simulink model "MLP_networks"  (Simulink 7.7)
settings: Solver=ode45  StartTime=0.0  StopTime=10.0  RelTol=1e-3
libraries: neural x1629
(part 13 of 39)

== system MLP_networks/net_col_c_d_2_4/Layer 2/LW{2,1} ==
  "ad{2,1}" : Inport  PortDimensions=30
      mask Display: e = 0.06;c1 = [120 230 180]/255;c2 = ([120 230 180]+0)/(256+128);c3 = ([120 230 180]+128)/(256+128);patch([0 1 1 0],[0 0 1 1],c1);patch([0 1 1 1-e 1-e 0+e],[0 0 1 1-e 0+e 0+e],c2);patch([0 0 1 1-e 0+e 0+e],[0 1 1 1-e 1-e 0+e],c3);plot([0 1 1 0 0],[0 0 1 1 0]);
  "IW{2,1}(1,:)'" : Constant  Value=[-0.086739905279401591;-0.34352499863211877;0.41397198976248467;0.43609623522289326;0.083435443764242001;0.19327035793616087;-0.27874403632422867;-0.11777803771657309;-0.023646706701705794;0.32594090440830897;-0.12873398528261154;0.33611135005815379;0.40852985787112106;-0.33466057721896658;-0.052474886443023012;0.43264924815576428;0.12741649927597465;0.03311259969224789;-0.19344074611037179;0.24350359634959076;-0.45438070656869112;0.40836563164644157;0.4762716734952942;-0.27838513598564113;-0.065634489210694244;-0.29128069108023635;0.25511712952102317;-0.46499974373678382;-0.0088992625430886971;0.13908009278308667]
      mask Display: e = 0.06;c1 = [120 150 230]/255;c2 = ([120 150 230]+0)/383;c3 = ([120 150 230]+128)/383;patch([0 1 1 0],[0 0 1 1],c1);patch([0 1 1 1-e 1-e 0+e],[0 0 1 1-e 0+e 0+e],c2);patch([0 0 1 1-e 0+e 0+e],[0 1 1 1-e 1-e 0+e],c3);plot([0 1 1 0 0],[0 0 1 1 0]);disp('weights');
  "IW{2,1}(10,:)'" : Constant  Value=[-0.36729620765024679;0.0050898962860818709;-0.0468691936394676;0.1253497976658039;0.47105014411088103;0.0033716376305642725;-0.41138077394803518;-0.32349762312197461;0.39546656477867215;-0.22070804075098249;0.042861658999594557;-0.12681144224424798;-0.25039111248890011;-0.3712654210908593;0.56958995394778955;-0.044483129058483888;-0.34197575262972091;0.17028025717551185;0.1085468634386007;0.14691948303331084;-0.19893228667253338;0.43968182733407096;-0.53408102802366886;0.17496913310039999;0.097757521509979323;0.33217818846497571;-0.045631385768622072;-0.37542745057039434;0.33335878174126277;-0.068873205774028126]
      mask Display: e = 0.06;c1 = [120 150 230]/255;c2 = ([120 150 230]+0)/383;c3 = ([120 150 230]+128)/383;patch([0 1 1 0],[0 0 1 1],c1);patch([0 1 1 1-e 1-e 0+e],[0 0 1 1-e 0+e 0+e],c2);patch([0 0 1 1-e 0+e 0+e],[0 1 1 1-e 1-e 0+e],c3);plot([0 1 1 0 0],[0 0 1 1 0]);disp('weights');
  "IW{2,1}(11,:)'" : Constant  Value=[-0.21023796895427466;0.21178254562760829;-0.1516673968740547;0.2773361318766529;0.012215682673962412;-0.48546667397653748;-0.18369601082146786;-0.26072759710949656;-0.053448210306775074;0.20320759307683936;0.15049891040467875;0.10455567206696842;0.4429239128696621;-0.20191752051219272;0.29857936146071512;0.48716984305870775;-0.21868844150185676;0.39089943245601361;-0.38722549529227124;0.20420721060355676;-0.58146629375206382;-0.14308677037043016;0.092893812514471041;-0.30523259519614931;-0.29641244502780845;0.055601417546032407;-0.14166216047879499;0.39149809987544448;0.3731245822311216;-0.083752309554754018]
      mask Display: e = 0.06;c1 = [120 150 230]/255;c2 = ([120 150 230]+0)/383;c3 = ([120 150 230]+128)/383;patch([0 1 1 0],[0 0 1 1],c1);patch([0 1 1 1-e 1-e 0+e],[0 0 1 1-e 0+e 0+e],c2);patch([0 0 1 1-e 0+e 0+e],[0 1 1 1-e 1-e 0+e],c3);plot([0 1 1 0 0],[0 0 1 1 0]);disp('weights');
  "IW{2,1}(12,:)'" : Constant  Value=[-0.22221752783866594;-0.463286764183786;0.32012275560695169;0.25096255632346381;0.0050231260198129787;-0.41543038790111159;-0.042578931985107822;-0.229325715588483;-0.094594039183964918;0.12192301882377349;-0.2291642495939753;0.34948087306916753;-0.22411941369390356;-0.25980901333444251;0.0099306671826360823;-0.21571241200028116;-0.3003090801392887;0.36235995289088319;0.41424763108456042;0.4549194867057913;-0.38526533593013734;-0.027743054382739805;-0.20900585233406158;-0.35337276927947708;0.11255897424267725;-0.039132173089780509;-0.42824103440953348;0.44315723034418508;0.084105476144599511;0.37576155528745614]
      mask Display: e = 0.06;c1 = [120 150 230]/255;c2 = ([120 150 230]+0)/383;c3 = ([120 150 230]+128)/383;patch([0 1 1 0],[0 0 1 1],c1);patch([0 1 1 1-e 1-e 0+e],[0 0 1 1-e 0+e 0+e],c2);patch([0 0 1 1-e 0+e 0+e],[0 1 1 1-e 1-e 0+e],c3);plot([0 1 1 0 0],[0 0 1 1 0]);disp('weights');
  "IW{2,1}(13,:)'" : Constant  Value=[0.26664690956162634;0.18588211338743232;-0.51074478099671949;-0.23272464385698416;-0.11789865989217188;0.33770596273549025;-0.41543902149946016;-0.20325083039795819;0.21359489198140075;0.23771981850878229;-0.10782260011209335;-0.4560526783866341;-0.49243186311351428;0.35164195674675991;0.091680564545084595;-0.1416316671420981;0.090346906082689124;-0.26101314139369514;-0.070749610911415614;-0.40337304681422642;0.11262128161825263;-0.27525094149576945;-0.12145424331596209;-0.3151042810855188;-0.12176588049624475;-0.40594084401160607;0.40726344059532144;-0.13387975813296663;0.48118452093616576;0.27020875321167304]
      mask Display: e = 0.06;c1 = [120 150 230]/255;c2 = ([120 150 230]+0)/383;c3 = ([120 150 230]+128)/383;patch([0 1 1 0],[0 0 1 1],c1);patch([0 1 1 1-e 1-e 0+e],[0 0 1 1-e 0+e 0+e],c2);patch([0 0 1 1-e 0+e 0+e],[0 1 1 1-e 1-e 0+e],c3);plot([0 1 1 0 0],[0 0 1 1 0]);disp('weights');
  "IW{2,1}(14,:)'" : Constant  Value=[0.34980934949483533;0.1234860655908767;0.41357778903144787;0.052540691627614988;0.25997646810356406;0.019550504650392903;-0.41112577725337546;-0.004004284700734397;0.20936217792212469;0.33508267363697175;-0.20605229449470713;0.30248198819108618;0.15830807524143486;-0.25625975309585886;-0.28171785254204545;0.39217753159778523;-0.39365391187201221;0.34365095949680785;0.179703187893896;0.39471168575822613;0.0051157792018336453;-0.09392142748098764;0.24890008564234903;0.27724910625266452;0.3897128187753453;0.43225990952346627;-0.4134253832902795;0.34873671936583894;-0.16432440790350927;-0.26930883733609756]
      mask Display: e = 0.06;c1 = [120 150 230]/255;c2 = ([120 150 230]+0)/383;c3 = ([120 150 230]+128)/383;patch([0 1 1 0],[0 0 1 1],c1);patch([0 1 1 1-e 1-e 0+e],[0 0 1 1-e 0+e 0+e],c2);patch([0 0 1 1-e 0+e 0+e],[0 1 1 1-e 1-e 0+e],c3);plot([0 1 1 0 0],[0 0 1 1 0]);disp('weights');
  "IW{2,1}(15,:)'" : Constant  Value=[0.10756034167331048;0.027268277800464581;0.23872494323237675;-0.26516481299813138;0.26000758623086434;-0.39846704436064129;-0.27015200960985691;-0.44604290248752793;0.42864135743800169;-0.4469329110749522;0.16848395781183378;-0.051220464237963677;0.086400763208768563;-0.10129868161474533;-0.026199243651805027;0.30436336508280776;-0.25002859827495977;-0.0072896443892497232;0.35355014668734541;0.37370190785436924;0.26582471435491495;-0.043249001392198672;0.44844689361690387;0.35439045498470667;0.21055831758031823;-0.27598099185526553;-0.35847563137517258;0.33563489845674022;0.3657385019059855;0.33310742263125259]
      mask Display: e = 0.06;c1 = [120 150 230]/255;c2 = ([120 150 230]+0)/383;c3 = ([120 150 230]+128)/383;patch([0 1 1 0],[0 0 1 1],c1);patch([0 1 1 1-e 1-e 0+e],[0 0 1 1-e 0+e 0+e],c2);patch([0 0 1 1-e 0+e 0+e],[0 1 1 1-e 1-e 0+e],c3);plot([0 1 1 0 0],[0 0 1 1 0]);disp('weights');
  "IW{2,1}(16,:)'" : Constant  Value=[-0.22297684824986103;-0.35714462966301846;0.48875156904773898;-0.04051019970576434;0.41685592475144728;-0.12244765379847856;-0.40779118540112924;0.023197515559235875;-0.045272172969816532;-0.023956146090705222;-0.44229605346214801;-0.10538638233096333;-0.30887898599700275;-0.40889553293161374;0.071952147052590343;-0.48675313221945821;-0.35492176719265267;-0.13320271136704864;0.25380506446655143;0.19576911876540612;0.15700698328941776;0.48317096404336252;0.31386156255509157;-0.29817432668524568;-0.23166046191463932;0.2076614117377503;-0.065995897941546824;-0.4446390086503117;0.10384621552539763;-0.10499763342719416]
      mask Display: e = 0.06;c1 = [120 150 230]/255;c2 = ([120 150 230]+0)/383;c3 = ([120 150 230]+128)/383;patch([0 1 1 0],[0 0 1 1],c1);patch([0 1 1 1-e 1-e 0+e],[0 0 1 1-e 0+e 0+e],c2);patch([0 0 1 1-e 0+e 0+e],[0 1 1 1-e 1-e 0+e],c3);plot([0 1 1 0 0],[0 0 1 1 0]);disp('weights');
  "IW{2,1}(17,:)'" : Constant  Value=[-0.20818659317735247;0.37291404688386326;-0.066412472318293309;0.23880592375907964;-0.17470240698411357;0.36274967181515411;-0.29500641736352323;0.3612460607052741;0.35349882887855227;0.50867004947603289;-0.24957816422824536;-0.37050881703534111;-0.17894190937801782;-0.4020952164867897;0.16763586618568879;-0.34269716360850005;0.31470217864282929;0.16211539237220335;0.35180618314252515;-0.052516647446877403;0.050581096159848335;0.039637997646489689;-0.2790044063742475;0.21372505912316375;0.087182966437931317;0.24205750316420507;-0.49727888668810799;-0.0062618082043166736;-0.66180921273073823;-0.15908637712630638]
      mask Display: e = 0.06;c1 = [120 150 230]/255;c2 = ([120 150 230]+0)/383;c3 = ([120 150 230]+128)/383;patch([0 1 1 0],[0 0 1 1],c1);patch([0 1 1 1-e 1-e 0+e],[0 0 1 1-e 0+e 0+e],c2);patch([0 0 1 1-e 0+e 0+e],[0 1 1 1-e 1-e 0+e],c3);plot([0 1 1 0 0],[0 0 1 1 0]);disp('weights');
  "IW{2,1}(18,:)'" : Constant  Value=[-0.063784427387764658;-0.32883070779687101;-0.48245120779581252;0.39650567321388691;-0.44937991772281205;0.01898057625759408;-0.12935469257041271;0.39546243145334697;-0.22112563100831639;0.38159471583348348;0.47658380504876108;0.29114272831383531;0.081150065748367251;-0.35952532056727365;0.43105590479120115;0.36632351247334227;0.088108073808608592;-0.37722671859528067;0.12912619522745261;0.23488410715253483;0.10081022555742715;0.11318476809914328;0.37249559297773699;0.22920497316165944;-0.089689746006884327;-0.053868567690606883;-0.37766729562412882;-0.35274036741954445;0.073527138309710388;-0.10041159535850687]
      mask Display: e = 0.06;c1 = [120 150 230]/255;c2 = ([120 150 230]+0)/383;c3 = ([120 150 230]+128)/383;patch([0 1 1 0],[0 0 1 1],c1);patch([0 1 1 1-e 1-e 0+e],[0 0 1 1-e 0+e 0+e],c2);patch([0 0 1 1-e 0+e 0+e],[0 1 1 1-e 1-e 0+e],c3);plot([0 1 1 0 0],[0 0 1 1 0]);disp('weights');
  "IW{2,1}(19,:)'" : Constant  Value=[0.19336196700834571;0.26744725560522559;-0.12860710197058553;0.31928174667930265;-0.070050044733280872;0.23283023634842093;0.30818323009661364;0.22289340702256244;-0.040112984385321182;0.46550220777364704;-0.35005738655757873;0.47597538337899226;-0.44170921923744139;-0.26572842897223375;-0.34489183248480759;0.18140277900820642;0.28607657081867038;0.086576963143464039;-0.3072812531424518;-0.034491965720857221;-0.39374044579926959;-0.18234841076921057;-0.35726304605837306;0.52328133768006635;0.21393030940681942;-0.11424070367808993;0.023196839579096535;0.15293831083094575;-0.30406146637276343;0.42953594576905829]
      mask Display: e = 0.06;c1 = [120 150 230]/255;c2 = ([120 150 230]+0)/383;c3 = ([120 150 230]+128)/383;patch([0 1 1 0],[0 0 1 1],c1);patch([0 1 1 1-e 1-e 0+e],[0 0 1 1-e 0+e 0+e],c2);patch([0 0 1 1-e 0+e 0+e],[0 1 1 1-e 1-e 0+e],c3);plot([0 1 1 0 0],[0 0 1 1 0]);disp('weights');
  "IW{2,1}(2,:)'" : Constant  Value=[-0.31476253520435571;-0.1138264490805047;-0.45036209335075572;0.2714809849441942;-0.18735671368056603;0.43408018666630871;-0.071620807727931404;0.048980335818204206;0.43751144967020755;0.020604521452307876;-0.10660971195039906;-0.3560330087569426;0.020071737319517006;-0.18091744791693601;0.40865545415885268;0.44681513013327728;0.38130042131451752;-0.23103110817028119;-0.42668382247905429;-0.39432400289217451;-0.22914394412555436;0.34667621785082403;-0.20755805619700282;0.057989851918950258;0.36069318624763025;0.34715274095295884;0.24150077728754232;0.2229140129936108;0.1240409175129034;-0.16506729455336752]
      mask Display: e = 0.06;c1 = [120 150 230]/255;c2 = ([120 150 230]+0)/383;c3 = ([120 150 230]+128)/383;patch([0 1 1 0],[0 0 1 1],c1);patch([0 1 1 1-e 1-e 0+e],[0 0 1 1-e 0+e 0+e],c2);patch([0 0 1 1-e 0+e 0+e],[0 1 1 1-e 1-e 0+e],c3);plot([0 1 1 0 0],[0 0 1 1 0]);disp('weights');
  "IW{2,1}(20,:)'" : Constant  Value=[0.33658701609073133;-0.17880093932274299;0.28437477283972262;0.39176322624983256;0.34816982312398603;-0.27806344079324408;-0.13224436335612005;0.23658674697646723;0.31463988161876533;0.23333367558291757;-0.20140728285472401;0.38983013905004149;-0.30351607692150379;-0.28449349935494206;-0.20626698506988783;-0.35004568799273844;-0.12100694505081969;0.21073444675825728;0.4293641950214887;-0.079932739921778573;-0.16946655759443563;-0.41523238613031477;-0.22719246897086262;0.11304598071208617;-0.1468262990874139;-0.50528490331397169;-0.43436092951156996;-0.40874554765229931;-0.15439640651095748;-0.10139444109459227]
      mask Display: e = 0.06;c1 = [120 150 230]/255;c2 = ([120 150 230]+0)/383;c3 = ([120 150 230]+128)/383;patch([0 1 1 0],[0 0 1 1],c1);patch([0 1 1 1-e 1-e 0+e],[0 0 1 1-e 0+e 0+e],c2);patch([0 0 1 1-e 0+e 0+e],[0 1 1 1-e 1-e 0+e],c3);plot([0 1 1 0 0],[0 0 1 1 0]);disp('weights');
  "IW{2,1}(21,:)'" : Constant  Value=[0.18698793822477749;0.44710802080556572;0.055362238215656438;-0.10315370156659233;-0.093547650109901181;0.48144329663092722;-0.3487454699215734;-0.3357544725505629;-0.52892778597397039;-0.15570016555093408;0.019344232566923886;-0.057459364801196039;-0.10882588337634393;-0.13026152839250427;0.31546914479780114;-0.54184132761413528;-0.20814735027442335;-0.50581397740701151;0.066142940955517926;-0.073780813119728506;-0.019554590542029657;0.3076647815515357;-0.51496038974850633;-0.20453340312828328;0.46321035495375734;0.12406975452781493;-0.025668149130415988;-0.16131670207754562;0.40620666634841929;-0.27237136393892403]
      mask Display: e = 0.06;c1 = [120 150 230]/255;c2 = ([120 150 230]+0)/383;c3 = ([120 150 230]+128)/383;patch([0 1 1 0],[0 0 1 1],c1);patch([0 1 1 1-e 1-e 0+e],[0 0 1 1-e 0+e 0+e],c2);patch([0 0 1 1-e 0+e 0+e],[0 1 1 1-e 1-e 0+e],c3);plot([0 1 1 0 0],[0 0 1 1 0]);disp('weights');
  "IW{2,1}(22,:)'" : Constant  Value=[-0.30183550782893204;0.18593285110881588;0.051690249772538249;0.42467534385490119;0.12917866311309761;-0.46077057472685201;0.023141069862614577;0.14345569870191224;-0.063414483521242584;0.48237058045684522;-0.055378234308140824;0.29182892206326488;0.42334775055828106;0.33457671039397663;0.43955355934047158;-0.0030498102862665721;0.34715523973677864;-0.37986667441238248;0.29783656860234109;0.12222242933619888;-0.044754535324555048;0.42544662656884691;-0.16407975067525937;-0.15912099798763263;-0.45811143300484625;-0.39655212784155747;0.31857894815139959;-0.23994535950314261;0.23029394329595129;0.10679840935171044]
      mask Display: e = 0.06;c1 = [120 150 230]/255;c2 = ([120 150 230]+0)/383;c3 = ([120 150 230]+128)/383;patch([0 1 1 0],[0 0 1 1],c1);patch([0 1 1 1-e 1-e 0+e],[0 0 1 1-e 0+e 0+e],c2);patch([0 0 1 1-e 0+e 0+e],[0 1 1 1-e 1-e 0+e],c3);plot([0 1 1 0 0],[0 0 1 1 0]);disp('weights');
  "IW{2,1}(23,:)'" : Constant  Value=[0.053371052201615247;-0.49742073003002413;-0.3599435655909598;0.16330570695765617;-0.41532433512319111;0.09863006949822134;-0.29326825977264376;0.30729900401793153;-0.065949061443200174;0.11198886134314458;0.36820832074642851;-0.24578993140959082;-0.15348153563585035;0.48631579535407221;0.13138601761928562;0.1266852664445573;0.14448148795735102;0.51816404532104388;0.21273550099709346;0.40532426732531829;0.14530829635166378;-0.37547464479146891;-0.39977913170225465;-0.17169438892309066;0.053399449589075901;0.36049043906111888;-0.18142893811318006;0.42052136186239569;0.18973264143336227;0.0041478850787327456]
      mask Display: e = 0.06;c1 = [120 150 230]/255;c2 = ([120 150 230]+0)/383;c3 = ([120 150 230]+128)/383;patch([0 1 1 0],[0 0 1 1],c1);patch([0 1 1 1-e 1-e 0+e],[0 0 1 1-e 0+e 0+e],c2);patch([0 0 1 1-e 0+e 0+e],[0 1 1 1-e 1-e 0+e],c3);plot([0 1 1 0 0],[0 0 1 1 0]);disp('weights');
  "IW{2,1}(24,:)'" : Constant  Value=[0.20516641930919408;-0.13518158187186338;0.0031559816953125831;0.18139980194621383;-0.54341365942738007;0.33949462411693088;0.10313907071790988;0.31393660081584912;0.11321227617715977;0.045980862742651681;0.27200974181943832;0.67565470147675843;-0.14522217595114961;0.51602354093719782;-0.14943402842186573;0.58352681264601935;-0.10609970694290385;-0.0058408385127818952;-0.27600492769484047;-0.068484010904123274;0.098456691211598016;-0.17902535749425891;-0.00037140347666213828;-0.23887433643879744;-0.057275554320067604;-0.50549685308164283;0.46414337205761558;0.10624528725808427;0.10579439676794743;0.15549185179355696]
      mask Display: e = 0.06;c1 = [120 150 230]/255;c2 = ([120 150 230]+0)/383;c3 = ([120 150 230]+128)/383;patch([0 1 1 0],[0 0 1 1],c1);patch([0 1 1 1-e 1-e 0+e],[0 0 1 1-e 0+e 0+e],c2);patch([0 0 1 1-e 0+e 0+e],[0 1 1 1-e 1-e 0+e],c3);plot([0 1 1 0 0],[0 0 1 1 0]);disp('weights');
  "IW{2,1}(25,:)'" : Constant  Value=[0.34729406478959007;0.24899528893076581;0.38975618702404735;-0.43370060705451807;0.43967599939440211;0.24714052363443123;-0.23516138628203193;0.27112310701103942;0.30747614819565189;-0.25901471912936047;0.066960381916171249;0.021109088740329799;0.36800329396956483;-0.33773092533269283;0.16585516170887771;-0.39913557490327317;0.422381088012171;0.38751406788119919;-0.28623287820901655;-0.18588164855613096;0.16437778958045182;0.33801033214529363;-0.14353924983108626;-0.27136982002342719;-0.18588379207432654;-0.19026604050441728;0.43711302651380946;0.082818735914955685;0.10823163927324558;0.17381563706576]
      mask Display: e = 0.06;c1 = [120 150 230]/255;c2 = ([120 150 230]+0)/383;c3 = ([120 150 230]+128)/383;patch([0 1 1 0],[0 0 1 1],c1);patch([0 1 1 1-e 1-e 0+e],[0 0 1 1-e 0+e 0+e],c2);patch([0 0 1 1-e 0+e 0+e],[0 1 1 1-e 1-e 0+e],c3);plot([0 1 1 0 0],[0 0 1 1 0]);disp('weights');
  "IW{2,1}(26,:)'" : Constant  Value=[0.39572013934362721;0.21877832829196214;-0.15198346332651508;0.42066807388437649;0.31599505644468512;0.15381761781263398;0.14191037298792222;-0.025831073713321617;-0.15017548056642216;0.094845571844094187;-0.46918736211706985;-0.24436647216383825;0.14124572797964732;-0.27098572544577526;-0.48977172048525852;-0.17053071487204099;-0.21764468329733291;0.55221642220574907;-0.48813591066651452;-0.14388962884454987;0.21413565468843948;0.01795983414699797;0.3500296082403242;-0.046075493068468559;0.023259972562694051;-0.16960957564902857;0.34946590680847733;-0.32493567344175694;-0.79675058574351276;-0.040157404112677854]
      mask Display: e = 0.06;c1 = [120 150 230]/255;c2 = ([120 150 230]+0)/383;c3 = ([120 150 230]+128)/383;patch([0 1 1 0],[0 0 1 1],c1);patch([0 1 1 1-e 1-e 0+e],[0 0 1 1-e 0+e 0+e],c2);patch([0 0 1 1-e 0+e 0+e],[0 1 1 1-e 1-e 0+e],c3);plot([0 1 1 0 0],[0 0 1 1 0]);disp('weights');
  "IW{2,1}(27,:)'" : Constant  Value=[0.32534994644003057;-0.41642829816325938;0.011570065792549176;-0.29786476644532855;0.45159915073304424;0.10977347223909036;0.41951308631372519;-0.2786677260959099;0.048270898093343499;0.40469287452714314;0.090762209641503638;0.30832948458024156;-0.44497998682067447;0.027023963167830067;0.43475271255433806;-0.31194882171522414;0.071104069846153389;-0.1218211168369496;-0.21603208889454797;0.085642327106287178;0.27138365529309416;0.17611522401418517;-0.42549139891614307;0.28814499726038512;0.11144377930775609;0.36334535252351047;0.030079906968749848;0.38238151675859983;-0.21145432284486562;0.3676888129471772]
      mask Display: e = 0.06;c1 = [120 150 230]/255;c2 = ([120 150 230]+0)/383;c3 = ([120 150 230]+128)/383;patch([0 1 1 0],[0 0 1 1],c1);patch([0 1 1 1-e 1-e 0+e],[0 0 1 1-e 0+e 0+e],c2);patch([0 0 1 1-e 0+e 0+e],[0 1 1 1-e 1-e 0+e],c3);plot([0 1 1 0 0],[0 0 1 1 0]);disp('weights');
  "IW{2,1}(28,:)'" : Constant  Value=[0.31509177300629926;0.14815248646653595;-0.2919124620695272;-0.4226568342460717;0.01553006383430215;0.17892296749635364;0.11079692958996719;0.096954504617871112;0.35243713326217668;0.17429482045049752;-0.52681042435863579;0.1189292096159086;-0.45378395170713492;0.41630627903960127;-0.43334391801673883;0.221199296666788;0.016586271003795429;-0.29375825107966386;-0.15602138806451321;0.27080779037297553;0.23092082963007024;0.34299541873533396;0.24829059293099975;-0.11178790671518112;0.37788202555986866;-0.30145460796278811;0.026090114181624179;-0.01542263523111944;-0.47761037085155578;0.31640852167676409]
      mask Display: e = 0.06;c1 = [120 150 230]/255;c2 = ([120 150 230]+0)/383;c3 = ([120 150 230]+128)/383;patch([0 1 1 0],[0 0 1 1],c1);patch([0 1 1 1-e 1-e 0+e],[0 0 1 1-e 0+e 0+e],c2);patch([0 0 1 1-e 0+e 0+e],[0 1 1 1-e 1-e 0+e],c3);plot([0 1 1 0 0],[0 0 1 1 0]);disp('weights');
  "IW{2,1}(29,:)'" : Constant  Value=[-0.25545162937697963;-0.25345640169393796;-0.072187848608269406;-0.31981528383242347;0.22688747248048238;0.016624939072259134;0.18821201366204474;0.17975496643804476;0.22182508310042173;0.22140298338907391;0.04616961859607558;0.44961522371237017;-0.27007625648999789;0.036199737266536858;-0.31033437050418688;0.50191286269037638;0.36693439377732634;0.38462614275662821;-0.34399498571882309;-0.30884483554802933;0.34930816572361606;-0.39983100603452681;0.11547430161276866;0.031676633777204262;0.46420448374530771;0.072881930176759965;-0.51379118153392078;0.026704920440349875;0.19817974035145186;-0.15837739569374379]
      mask Display: e = 0.06;c1 = [120 150 230]/255;c2 = ([120 150 230]+0)/383;c3 = ([120 150 230]+128)/383;patch([0 1 1 0],[0 0 1 1],c1);patch([0 1 1 1-e 1-e 0+e],[0 0 1 1-e 0+e 0+e],c2);patch([0 0 1 1-e 0+e 0+e],[0 1 1 1-e 1-e 0+e],c3);plot([0 1 1 0 0],[0 0 1 1 0]);disp('weights');
  "IW{2,1}(3,:)'" : Constant  Value=[0.20791470698880146;-0.35147459161660466;0.16251561527311512;0.18068384160700443;-0.32012933851815295;0.10040390459823008;-0.25450004278317045;-0.55004306714329709;-0.17953992654907994;0.50142016798885369;0.19388814837504995;-0.57558212642281636;-0.44000700127006354;-0.020620085052794866;0.13449438434095745;0.15298036066838266;-0.30329518695363417;0.52248259377675599;-0.097644117202854153;-0.14344776725053776;0.11620338058491989;-0.13091188822745206;-0.36753669206193273;-0.056127523648647766;0.38108244624528742;-0.22220680571181917;-0.32560529568944463;0.34155073187854679;0.2740198786862536;0.36692196661375026]
      mask Display: e = 0.06;c1 = [120 150 230]/255;c2 = ([120 150 230]+0)/383;c3 = ([120 150 230]+128)/383;patch([0 1 1 0],[0 0 1 1],c1);patch([0 1 1 1-e 1-e 0+e],[0 0 1 1-e 0+e 0+e],c2);patch([0 0 1 1-e 0+e 0+e],[0 1 1 1-e 1-e 0+e],c3);plot([0 1 1 0 0],[0 0 1 1 0]);disp('weights');
  "IW{2,1}(30,:)'" : Constant  Value=[0.35133724217297468;-0.40144310755179119;-0.123816188538727;0.13501461692444083;-0.22386861846353476;-0.54848747166277256;-0.34140736497182478;-0.15298204686301042;0.20773511342421272;0.39517894286497673;-0.10624926490974719;-0.1804639807038742;0.0081221377490989285;-0.40062862717106534;-0.26413202307108036;0.20913209762848348;0.34124610314533921;-0.22746527754564308;0.043250804742566831;-0.37495543053121799;-0.23824428558657995;-0.12883971068677164;-0.10042385343760465;0.44883317354485952;0.47358116906029774;-0.17946122640242748;0.13516773263075868;0.50836936330348814;0.1616595353780389;0.18544387018013045]
      mask Display: e = 0.06;c1 = [120 150 230]/255;c2 = ([120 150 230]+0)/383;c3 = ([120 150 230]+128)/383;patch([0 1 1 0],[0 0 1 1],c1);patch([0 1 1 1-e 1-e 0+e],[0 0 1 1-e 0+e 0+e],c2);patch([0 0 1 1-e 0+e 0+e],[0 1 1 1-e 1-e 0+e],c3);plot([0 1 1 0 0],[0 0 1 1 0]);disp('weights');
  "IW{2,1}(31,:)'" : Constant  Value=[-0.19072607038306774;0.0018036307514540486;-0.4953964240309145;-0.061847140723814004;0.098287756157279138;0.35336181566066294;0.36939348668649025;-0.12419386513481664;0.25666984160845296;0.483545917074653;0.50369576084414591;0.14220775090891918;-0.05018010301479333;0.072750876768745545;-0.36112739686115425;0.54179891998336038;0.24337274489791302;0.23823620883315189;-0.22827299772039039;-0.022779613982744612;0.41288552477346019;0.16118633478119779;-0.45370449722072453;0.062194540032977273;0.011252531066492948;0.32939314694012617;-0.40237417247645701;0.027208821151308848;0.26477271837998356;-0.12804121454167405]
      mask Display: e = 0.06;c1 = [120 150 230]/255;c2 = ([120 150 230]+0)/383;c3 = ([120 150 230]+128)/383;patch([0 1 1 0],[0 0 1 1],c1);patch([0 1 1 1-e 1-e 0+e],[0 0 1 1-e 0+e 0+e],c2);patch([0 0 1 1-e 0+e 0+e],[0 1 1 1-e 1-e 0+e],c3);plot([0 1 1 0 0],[0 0 1 1 0]);disp('weights');
  "IW{2,1}(32,:)'" : Constant  Value=[0.4502734263643145;-0.11642585097845862;-0.41824840582007511;0.23721387308435984;0.30528144202757262;0.4134028608462279;-0.0064459057861856288;-0.35202249700738092;-0.44372073752373431;-0.0039987239173472581;-0.28642302929489294;-0.074740850463484762;0.20315463744205187;-0.26484765920428727;0.1870815706184262;-0.34566385979792968;0.22276433847201366;-0.27930940965665979;-0.15821577536788484;0.30280727717311667;-0.26841341019238035;0.045641895422698579;-0.45206391096580273;-0.38237736318509152;-0.42809026571481001;-0.40690699607408048;-0.30183694501274461;0.1984273371036552;0.27452300279277181;-0.14091162981366676]
      mask Display: e = 0.06;c1 = [120 150 230]/255;c2 = ([120 150 230]+0)/383;c3 = ([120 150 230]+128)/383;patch([0 1 1 0],[0 0 1 1],c1);patch([0 1 1 1-e 1-e 0+e],[0 0 1 1-e 0+e 0+e],c2);patch([0 0 1 1-e 0+e 0+e],[0 1 1 1-e 1-e 0+e],c3);plot([0 1 1 0 0],[0 0 1 1 0]);disp('weights');
  "IW{2,1}(33,:)'" : Constant  Value=[-0.41268246385026286;-0.079120679591981699;-0.25359870818272284;0.34268725352457979;-0.47347510355362321;-0.11016464012586072;0.14591017518403196;-0.38118158667382662;0.35560987453304987;0.32668665940123554;0.068886753730610942;-0.22116215831674615;0.36402450973391665;-0.45048920658265645;0.42771451770498531;-0.23360803915440473;0.14391309847501285;-0.088248037794645351;-0.052342111906455706;0.10766643851055042;0.092020441508780054;-0.26519804107971368;-0.18483379704589606;-0.40452038629829984;-0.41451018977306792;0.36275456448229504;0.3876279077581955;0.40070560331044225;-0.25846786547072348;0.18290179281854513]
      mask Display: e = 0.06;c1 = [120 150 230]/255;c2 = ([120 150 230]+0)/383;c3 = ([120 150 230]+128)/383;patch([0 1 1 0],[0 0 1 1],c1);patch([0 1 1 1-e 1-e 0+e],[0 0 1 1-e 0+e 0+e],c2);patch([0 0 1 1-e 0+e 0+e],[0 1 1 1-e 1-e 0+e],c3);plot([0 1 1 0 0],[0 0 1 1 0]);disp('weights');
  "IW{2,1}(34,:)'" : Constant  Value=[0.26458554722026689;-0.14083341967377108;0.26426606557715993;-0.35799487854237061;-0.12671910807629308;-0.38335510375252735;0.40076498033273666;-0.37790753942195504;0.21965558526959253;0.14508275111250124;0.39103081048016841;0.3570387341837894;-0.31835792840882088;0.24782372448200518;-0.31356502274635895;0.14700702022151749;0.43592824611169301;-0.14576134864896531;-0.28314466918174896;0.43874352934185151;-0.2911634380312812;-0.21275783319015867;-0.40201259274536572;0.036789213618181278;-0.36030255601872291;0.024881816643906048;-0.11844008090397237;0.23279047678228673;0.25528638844820795;-0.25416858231463757]
      mask Display: e = 0.06;c1 = [120 150 230]/255;c2 = ([120 150 230]+0)/383;c3 = ([120 150 230]+128)/383;patch([0 1 1 0],[0 0 1 1],c1);patch([0 1 1 1-e 1-e 0+e],[0 0 1 1-e 0+e 0+e],c2);patch([0 0 1 1-e 0+e 0+e],[0 1 1 1-e 1-e 0+e],c3);plot([0 1 1 0 0],[0 0 1 1 0]);disp('weights');
  "IW{2,1}(35,:)'" : Constant  Value=[0.14709850217691736;0.51431244311169944;-0.49529590283945074;-0.13884478915023282;-0.33270125896632446;0.4479055585945419;-0.34471176449324842;0.1104980976716211;0.43016998053170952;0.30829623171158077;-0.00067094059965810645;0.2093860214916296;-0.19136773567958917;-0.087537166192539095;-0.21632727454702744;0.11894873978528084;0.36774093181596434;-0.20707391273027947;-0.47860536455884567;0.45083169304522047;-0.38771308084372835;0.18267762130396781;-0.1382943938610286;0.19899812616135293;-0.001997470000718374;-0.037026143400154504;-0.22308570722191687;-0.38502969617913624;0.0039339675119745956;0.20699041496582496]
      mask Display: e = 0.06;c1 = [120 150 230]/255;c2 = ([120 150 230]+0)/383;c3 = ([120 150 230]+128)/383;patch([0 1 1 0],[0 0 1 1],c1);patch([0 1 1 1-e 1-e 0+e],[0 0 1 1-e 0+e 0+e],c2);patch([0 0 1 1-e 0+e 0+e],[0 1 1 1-e 1-e 0+e],c3);plot([0 1 1 0 0],[0 0 1 1 0]);disp('weights');
  "IW{2,1}(36,:)'" : Constant  Value=[0.38988623118316468;-0.22597432812402868;0.060120511520675275;-0.17092612605555274;-0.28132926813541326;0.096404141878804431;0.1916241595895164;0.057572950676559251;-0.084444190455332524;0.50110425889936416;-0.16811660816492963;0.38869266200690133;0.42925017904820167;0.4743155363757246;0.1495103732197616;-0.032613730169453008;0.036150512293197969;-0.30428003626854494;0.25861263973834742;-0.13530899943219979;-0.38886773117711138;0.40220797375780509;0.27728677367935806;0.46919995980103857;-0.14845126494883523;0.30836423874050484;-0.21336282261843056;-0.42626758746633786;-0.093286506167299638;-0.39787707258605037]
      mask Display: e = 0.06;c1 = [120 150 230]/255;c2 = ([120 150 230]+0)/383;c3 = ([120 150 230]+128)/383;patch([0 1 1 0],[0 0 1 1],c1);patch([0 1 1 1-e 1-e 0+e],[0 0 1 1-e 0+e 0+e],c2);patch([0 0 1 1-e 0+e 0+e],[0 1 1 1-e 1-e 0+e],c3);plot([0 1 1 0 0],[0 0 1 1 0]);disp('weights');
  "IW{2,1}(37,:)'" : Constant  Value=[-0.4639589987613339;0.40265599828641663;-0.1012083229193006;0.10791809194053954;-0.012295815732515815;0.19557144087120493;0.23998687313820111;0.38458770038796825;-0.32184788735486408;-0.078463200939442451;-0.018161380981613632;0.2009028677518547;-0.39448576802987545;-0.026995884108561779;0.47684260080330315;-0.37304301141296597;0.29408965640335977;-0.05473477922646184;0.29868858269369442;-0.37335741638873166;0.1655622343493405;0.1736046790296569;-0.40132426136540189;0.22198289548752922;0.16226915725241658;-0.27594559826662063;0.039159711964272301;-0.34644717329830549;-0.54412412728372872;-0.45085970426782657]
      mask Display: e = 0.06;c1 = [120 150 230]/255;c2 = ([120 150 230]+0)/383;c3 = ([120 150 230]+128)/383;patch([0 1 1 0],[0 0 1 1],c1);patch([0 1 1 1-e 1-e 0+e],[0 0 1 1-e 0+e 0+e],c2);patch([0 0 1 1-e 0+e 0+e],[0 1 1 1-e 1-e 0+e],c3);plot([0 1 1 0 0],[0 0 1 1 0]);disp('weights');
  "IW{2,1}(38,:)'" : Constant  Value=[-0.37429037305154383;-0.034206705161056776;-0.4161677662377492;0.49833872357293946;-0.4086804372356671;-0.07301675456432058;-0.040603021485009987;0.44287099711723266;-0.41651016308601019;0.19267069866514025;-0.16382918177513989;0.071149679318055159;0.22176216468118753;0.34535219152746727;0.25368738217667053;-0.41558090893805122;-0.091879890611968079;-0.27836191433279617;0.050007549793882708;0.12131145678897313;-0.062264211985549871;-0.18661082738229834;0.052380828795337835;0.36255817627509274;0.44418592364323778;-0.35038134509608965;0.33236359573161273;0.30945987094777039;0.2463457194001237;0.029590173850392795]
      mask Display: e = 0.06;c1 = [120 150 230]/255;c2 = ([120 150 230]+0)/383;c3 = ([120 150 230]+128)/383;patch([0 1 1 0],[0 0 1 1],c1);patch([0 1 1 1-e 1-e 0+e],[0 0 1 1-e 0+e 0+e],c2);patch([0 0 1 1-e 0+e 0+e],[0 1 1 1-e 1-e 0+e],c3);plot([0 1 1 0 0],[0 0 1 1 0]);disp('weights');
  "IW{2,1}(39,:)'" : Constant  Value=[-0.38529969820681731;-0.059674753731825028;-0.18025585793909021;0.48908167944049941;0.23136895782201464;0.2108574943827774;0.30273126789184113;0.19311046877985136;-0.44643155501147858;-0.49132952381431633;-0.31702242031783012;0.28878149498439115;-0.090488165212609162;0.15612809467264263;0.074351485219160615;-0.42270559191614049;0.19256973883304085;-0.26157280426424107;-0.13578338417934596;-0.1956289305276758;0.36885128636506836;0.1740089288591066;0.22341284228424213;-0.15504936919521459;-0.17380529904896855;0.27291353679079683;-0.092979025827366585;-0.37760996249470391;-0.075859646127589483;-0.55592057957484076]
      mask Display: e = 0.06;c1 = [120 150 230]/255;c2 = ([120 150 230]+0)/383;c3 = ([120 150 230]+128)/383;patch([0 1 1 0],[0 0 1 1],c1);patch([0 1 1 1-e 1-e 0+e],[0 0 1 1-e 0+e 0+e],c2);patch([0 0 1 1-e 0+e 0+e],[0 1 1 1-e 1-e 0+e],c3);plot([0 1 1 0 0],[0 0 1 1 0]);disp('weights');
  "IW{2,1}(4,:)'" : Constant  Value=[-0.092956610415413796;0.34069093986139942;-0.44956075646272292;0.35379876954456851;0.32975355189756683;0.10143837421044716;0.15773004176513908;-0.034082348796094938;-0.15988067982044385;0.33388394655029796;-0.10348211221488647;-0.22907988801225129;0.12726366783455098;-0.29303935272358939;-0.46326418107886624;0.11394962475047377;-0.42812223370604319;-0.3637929170673293;0.24667116095762845;-0.45308891597071183;0.25525017353847679;-0.39173586668797394;0.16247762962275955;0.063114929945691386;0.35501430427057057;0.22512116677866448;0.333243574696579;0.37145828794428304;0.023604183868472801;0.20615541408084995]
      mask Display: e = 0.06;c1 = [120 150 230]/255;c2 = ([120 150 230]+0)/383;c3 = ([120 150 230]+128)/383;patch([0 1 1 0],[0 0 1 1],c1);patch([0 1 1 1-e 1-e 0+e],[0 0 1 1-e 0+e 0+e],c2);patch([0 0 1 1-e 0+e 0+e],[0 1 1 1-e 1-e 0+e],c3);plot([0 1 1 0 0],[0 0 1 1 0]);disp('weights');
  "IW{2,1}(40,:)'" : Constant  Value=[0.16662393871729037;-0.43037330092297676;-0.047236313736522172;0.35321900256969724;0.10162747232591172;-0.36775165300013962;0.28534287203169445;-0.045423808480529994;0.40951255681762738;0.43323629374357636;-0.11745772382485413;0.26119280790061838;-0.24598202036727812;-0.30899553791441642;-0.080606304546670005;0.41943108934907086;-0.14021022576247949;-0.14638704678749076;-0.4431914759001167;0.3780210162195824;0.081391757470756276;0.063657044596717768;0.39817897156716264;-0.004892351028355499;-0.2635683681017334;0.054282611465783566;0.37057276519984284;-0.46061678979504217;-0.47128063206866866;0.015405056063258137]
      mask Display: e = 0.06;c1 = [120 150 230]/255;c2 = ([120 150 230]+0)/383;c3 = ([120 150 230]+128)/383;patch([0 1 1 0],[0 0 1 1],c1);patch([0 1 1 1-e 1-e 0+e],[0 0 1 1-e 0+e 0+e],c2);patch([0 0 1 1-e 0+e 0+e],[0 1 1 1-e 1-e 0+e],c3);plot([0 1 1 0 0],[0 0 1 1 0]);disp('weights');
  "IW{2,1}(5,:)'" : Constant  Value=[0.3852876191637496;0.23201511523175503;-0.28757062372467934;-0.47579185306563526;-0.00765372916228786;0.30658069771968138;-0.036168401959535496;0.32614354125407313;-0.069004179483434291;-0.081446183786577725;0.52703607333162594;0.16041552931051245;0.35600177001426048;-0.11337050284613553;0.29873824858130599;-0.48589466589639674;0.027313618864292948;0.45265889522885905;-0.21053152986930956;-0.13525940807057601;-0.39222402914721405;-0.19434301260696266;-0.13786605091582871;-0.21116907132582965;0.05523395635190384;-0.38549329971129936;-0.34511667873048218;0.37292831399551979;0.27387161426599399;0.08621963851057346]
      mask Display: e = 0.06;c1 = [120 150 230]/255;c2 = ([120 150 230]+0)/383;c3 = ([120 150 230]+128)/383;patch([0 1 1 0],[0 0 1 1],c1);patch([0 1 1 1-e 1-e 0+e],[0 0 1 1-e 0+e 0+e],c2);patch([0 0 1 1-e 0+e 0+e],[0 1 1 1-e 1-e 0+e],c3);plot([0 1 1 0 0],[0 0 1 1 0]);disp('weights');
  "IW{2,1}(6,:)'" : Constant  Value=[-0.45750772983536359;-0.17445659048171108;-0.28669545104413863;0.13038934093308427;-0.11991569341950845;-0.4494913152234376;-0.052981379135312007;-0.033170279342111156;-0.002353927011433559;-0.44268108625602465;-0.38147716990283315;-0.11364894140336372;0.3467037662840598;0.11087182257766652;-0.11425983351831892;0.081078209531570009;0.42965254748193799;-0.12085605724190772;0.038895552398031254;-0.33870819428779098;-0.4324311438019699;-0.062649512791331033;0.29906300823930265;0.43701439682305998;0.269029639601852;-0.35253737351876646;-0.44782438666150243;-0.22850533491712985;0.41599537540661563;-0.17423697835570115]
      mask Display: e = 0.06;c1 = [120 150 230]/255;c2 = ([120 150 230]+0)/383;c3 = ([120 150 230]+128)/383;patch([0 1 1 0],[0 0 1 1],c1);patch([0 1 1 1-e 1-e 0+e],[0 0 1 1-e 0+e 0+e],c2);patch([0 0 1 1-e 0+e 0+e],[0 1 1 1-e 1-e 0+e],c3);plot([0 1 1 0 0],[0 0 1 1 0]);disp('weights');
  "IW{2,1}(7,:)'" : Constant  Value=[-0.26530518730858332;-0.16090258282752185;-0.015375359625756898;-0.30414556453790093;-0.1734833926188227;0.27353803647115604;0.21132010103132792;-0.26973139942436847;-0.26754182749394512;0.31801632658272083;-0.075931789545092221;0.24070200643722489;0.47151250420764101;-0.078232978062307737;0.35083475793033464;0.44920353299413179;-0.49006823190812571;0.30657699132242094;0.45629270891128704;-0.31646316698908111;-0.25923308505405751;-0.39633903485312733;0.10896221495391963;-0.18616461523471592;-0.15975292242784267;-0.40507974603359131;-0.12962508942914377;-0.17409256821708868;-0.40735381004505228;0.15449188929180915]
      mask Display: e = 0.06;c1 = [120 150 230]/255;c2 = ([120 150 230]+0)/383;c3 = ([120 150 230]+128)/383;patch([0 1 1 0],[0 0 1 1],c1);patch([0 1 1 1-e 1-e 0+e],[0 0 1 1-e 0+e 0+e],c2);patch([0 0 1 1-e 0+e 0+e],[0 1 1 1-e 1-e 0+e],c3);plot([0 1 1 0 0],[0 0 1 1 0]);disp('weights');
  "IW{2,1}(8,:)'" : Constant  Value=[-0.46244643557141279;0.30491196597952652;0.22902205677991813;0.45088175023581778;0.18314038627712004;0.030720201232387213;0.35272613401612796;-0.36610052195822679;-0.3796890085264637;-0.40861093374972302;0.083133673962969334;-0.34318852368837327;0.24168545822035342;0.028022255572662746;0.027738663986734934;0.24066403373787709;0.26896188176750796;-0.45202604259231227;-0.43258643292158544;0.36629464747689539;0.025023314934505998;-0.061194014009970779;-0.20494249168856835;-0.18369649438652808;-0.30322345097686304;-0.27596908662436692;-0.11915396984828107;-0.18844768865720316;-0.31155559631779106;0.26429822768702482]
      mask Display: e = 0.06;c1 = [120 150 230]/255;c2 = ([120 150 230]+0)/383;c3 = ([120 150 230]+128)/383;patch([0 1 1 0],[0 0 1 1],c1);patch([0 1 1 1-e 1-e 0+e],[0 0 1 1-e 0+e 0+e],c2);patch([0 0 1 1-e 0+e 0+e],[0 1 1 1-e 1-e 0+e],c3);plot([0 1 1 0 0],[0 0 1 1 0]);disp('weights');
  "IW{2,1}(9,:)'" : Constant  Value=[-0.40291521296009208;0.11457314683464705;-0.16573640361094341;-0.44427958669432221;-0.37362247949660876;-0.41912837165929673;-0.26445031332342195;0.40199133020761796;0.13845849691377995;-0.01839159323961418;-0.40216639956545369;0.34330692326089923;0.24649842726239329;-0.40708272072703305;-0.37937002881350917;-0.11917824039566538;0.10224911879708322;-0.31187952151595638;-0.23541470196887282;0.2454973615284923;0.24975608089579995;-0.033933123554616737;-0.067297584958124657;0.22251604624646168;-0.43260865465484827;-0.39509969990063126;-0.32012895106396078;0.13456488050977683;0.20264236619400111;0.067517862285206551]
      mask Display: e = 0.06;c1 = [120 150 230]/255;c2 = ([120 150 230]+0)/383;c3 = ([120 150 230]+128)/383;patch([0 1 1 0],[0 0 1 1],c1);patch([0 1 1 1-e 1-e 0+e],[0 0 1 1-e 0+e 0+e],c2);patch([0 0 1 1-e 0+e 0+e],[0 1 1 1-e 1-e 0+e],c3);plot([0 1 1 0 0],[0 0 1 1 0]);disp('weights');
  Mux : Mux  Inputs=40
      mask Display: e = 0.06;c1 = [120 150 230]/255;c2 = ([120 150 230]+0)/383;c3 = ([120 150 230]+128)/383;patch([0 1 1 0],[0 0 1 1],c1);patch([0 1 1 1-e 1-e 0+e],[0 0 1 1-e 0+e 0+e],c2);patch([0 0 1 1-e 0+e 0+e],[0 1 1 1-e 1-e 0+e],c3);plot([0 1 1 0 0],[0 0 1 1 0]);disp('Mux');
  dotprod{1..40} (40 alike) : neural/Weight Functions/dotprod  SystemSampleTime=-1
  "lz{2,1}" : Outport
      mask Display: e = 0.06;c1 = [120 230 180]/255;c2 = ([120 230 180]+0)/(256+128);c3 = ([120 230 180]+128)/(256+128);patch([0 1 1 0],[0 0 1 1],c1);patch([0 1 1 1-e 1-e 0+e],[0 0 1 1-e 0+e 0+e],c2);patch([0 0 1 1-e 0+e 0+e],[0 1 1 1-e 1-e 0+e],c3);plot([0 1 1 0 0],[0 0 1 1 0]);
  wires:
  "IW{2,1}(1,:)'"/1 -> dotprod1/1
  "ad{2,1}"/1 -> dotprod1/2, dotprod2/2, dotprod3/2, dotprod4/2, dotprod5/2, dotprod6/2, dotprod7/2, dotprod8/2, dotprod9/2, dotprod10/2, dotprod11/2, dotprod12/2, dotprod13/2, dotprod14/2, dotprod15/2, dotprod16/2, dotprod17/2, dotprod18/2, dotprod19/2, dotprod20/2, dotprod21/2, dotprod22/2, dotprod23/2, dotprod24/2, dotprod25/2, dotprod26/2, dotprod27/2, dotprod28/2, dotprod29/2, dotprod30/2, dotprod31/2, dotprod32/2, dotprod33/2, dotprod34/2, dotprod35/2, dotprod36/2, dotprod37/2, dotprod38/2, dotprod39/2, dotprod40/2
  dotprod1/1 -> Mux/1
  "IW{2,1}(2,:)'"/1 -> dotprod2/1
  dotprod2/1 -> Mux/2
  "IW{2,1}(3,:)'"/1 -> dotprod3/1
  dotprod3/1 -> Mux/3
  "IW{2,1}(4,:)'"/1 -> dotprod4/1
  dotprod4/1 -> Mux/4
  "IW{2,1}(5,:)'"/1 -> dotprod5/1
  dotprod5/1 -> Mux/5
  "IW{2,1}(6,:)'"/1 -> dotprod6/1
  dotprod6/1 -> Mux/6
  "IW{2,1}(7,:)'"/1 -> dotprod7/1
  dotprod7/1 -> Mux/7
  "IW{2,1}(8,:)'"/1 -> dotprod8/1
  dotprod8/1 -> Mux/8
  "IW{2,1}(9,:)'"/1 -> dotprod9/1
  dotprod9/1 -> Mux/9
  "IW{2,1}(10,:)'"/1 -> dotprod10/1
  dotprod10/1 -> Mux/10
  "IW{2,1}(11,:)'"/1 -> dotprod11/1
  dotprod11/1 -> Mux/11
  "IW{2,1}(12,:)'"/1 -> dotprod12/1
  dotprod12/1 -> Mux/12
  "IW{2,1}(13,:)'"/1 -> dotprod13/1
  dotprod13/1 -> Mux/13
  "IW{2,1}(14,:)'"/1 -> dotprod14/1
  dotprod14/1 -> Mux/14
  "IW{2,1}(15,:)'"/1 -> dotprod15/1
  dotprod15/1 -> Mux/15
  "IW{2,1}(16,:)'"/1 -> dotprod16/1
  dotprod16/1 -> Mux/16
  "IW{2,1}(17,:)'"/1 -> dotprod17/1
  dotprod17/1 -> Mux/17
  "IW{2,1}(18,:)'"/1 -> dotprod18/1
  dotprod18/1 -> Mux/18
  "IW{2,1}(19,:)'"/1 -> dotprod19/1
  dotprod19/1 -> Mux/19
  "IW{2,1}(20,:)'"/1 -> dotprod20/1
  dotprod20/1 -> Mux/20
  "IW{2,1}(21,:)'"/1 -> dotprod21/1
  dotprod21/1 -> Mux/21
  "IW{2,1}(22,:)'"/1 -> dotprod22/1
  dotprod22/1 -> Mux/22
  "IW{2,1}(23,:)'"/1 -> dotprod23/1
  dotprod23/1 -> Mux/23
  "IW{2,1}(24,:)'"/1 -> dotprod24/1
  dotprod24/1 -> Mux/24
  "IW{2,1}(25,:)'"/1 -> dotprod25/1
  dotprod25/1 -> Mux/25
  "IW{2,1}(26,:)'"/1 -> dotprod26/1
  dotprod26/1 -> Mux/26
  "IW{2,1}(27,:)'"/1 -> dotprod27/1
  dotprod27/1 -> Mux/27
  "IW{2,1}(28,:)'"/1 -> dotprod28/1
  dotprod28/1 -> Mux/28
  "IW{2,1}(29,:)'"/1 -> dotprod29/1
  dotprod29/1 -> Mux/29
  "IW{2,1}(30,:)'"/1 -> dotprod30/1
  dotprod30/1 -> Mux/30
  "IW{2,1}(31,:)'"/1 -> dotprod31/1
  dotprod31/1 -> Mux/31
  "IW{2,1}(32,:)'"/1 -> dotprod32/1
  dotprod32/1 -> Mux/32
  "IW{2,1}(33,:)'"/1 -> dotprod33/1
  dotprod33/1 -> Mux/33
  "IW{2,1}(34,:)'"/1 -> dotprod34/1
  dotprod34/1 -> Mux/34
  "IW{2,1}(35,:)'"/1 -> dotprod35/1
  dotprod35/1 -> Mux/35
  "IW{2,1}(36,:)'"/1 -> dotprod36/1
  dotprod36/1 -> Mux/36
  "IW{2,1}(37,:)'"/1 -> dotprod37/1
  dotprod37/1 -> Mux/37
  "IW{2,1}(38,:)'"/1 -> dotprod38/1
  dotprod38/1 -> Mux/38
  "IW{2,1}(39,:)'"/1 -> dotprod39/1
  dotprod39/1 -> Mux/39
  "IW{2,1}(40,:)'"/1 -> dotprod40/1
  dotprod40/1 -> Mux/40
  Mux/1 -> "lz{2,1}"/1

== system MLP_networks/net_col_c_d_2_4/Layer 3/Delays 1 ==
  "p{3}" : Inport  PortDimensions=40
      mask Display: e = 0.06;c1 = [120 230 180]/255;c2 = ([120 230 180]+0)/(256+128);c3 = ([120 230 180]+128)/(256+128);patch([0 1 1 0],[0 0 1 1],c1);patch([0 1 1 1-e 1-e 0+e],[0 0 1 1-e 0+e 0+e],c2);patch([0 0 1 1-e 0+e 0+e],[0 1 1 1-e 1-e 0+e],c3);plot([0 1 1 0 0],[0 0 1 1 0]);
  mux : Mux  Inputs=1
      mask Display: e = 0.06;c1 = [120 150 230]/255;c2 = ([120 150 230]+0)/383;c3 = ([120 150 230]+128)/383;patch([0 1 1 0],[0 0 1 1],c1);patch([0 1 1 1-e 1-e 0+e],[0 0 1 1-e 0+e 0+e],c2);patch([0 0 1 1-e 0+e 0+e],[0 1 1 1-e 1-e 0+e],c3);plot([0 1 1 0 0],[0 0 1 1 0]);disp('Mux')
  "pd{3,2}" : Outport
      mask Display: e = 0.06;c1 = [120 230 180]/255;c2 = ([120 230 180]+0)/(256+128);c3 = ([120 230 180]+128)/(256+128);patch([0 1 1 0],[0 0 1 1],c1);patch([0 1 1 1-e 1-e 0+e],[0 0 1 1-e 0+e 0+e],c2);patch([0 0 1 1-e 0+e 0+e],[0 1 1 1-e 1-e 0+e],c3);plot([0 1 1 0 0],[0 0 1 1 0]);
  wires:
  "p{3}"/1 -> mux/1
  mux/1 -> "pd{3,2}"/1

== system MLP_networks/net_col_c_d_2_4/Layer 3/LW{3,2} ==
  "ad{3,2}" : Inport  PortDimensions=40
      mask Display: e = 0.06;c1 = [120 230 180]/255;c2 = ([120 230 180]+0)/(256+128);c3 = ([120 230 180]+128)/(256+128);patch([0 1 1 0],[0 0 1 1],c1);patch([0 1 1 1-e 1-e 0+e],[0 0 1 1-e 0+e 0+e],c2);patch([0 0 1 1-e 0+e 0+e],[0 1 1 1-e 1-e 0+e],c3);plot([0 1 1 0 0],[0 0 1 1 0]);
  "IW{3,2}(1,:)'" : Constant  Value=[0.50496456486038965;0.23825228384982539;0.68095932916282409;0.56559176884793461;0.05998094366874894;-0.035051904629260951;-0.23988422668233272;0.2095821886518624;-0.13930646717495407;-0.80366286069142356;-0.67383188620344936;0.74942168871273351;0.68351579297820286;-0.25455944056747076;0.28331207265962954;-0.30530368024477361;-1.0329969673828463;-0.80146712320872737;0.21414310747924897;-0.2930800962455764;0.8853125821498653;0.39209370509137526;0.0063358829854075534;0.83313938853591818;0.74191805001744426;-1.0742930345471424;-0.015210286409165033;-0.65683839198243021;-0.87574518933712964;-0.58162065914238759;-0.084123130636696367;-0.72305573374756049;0.69656776594858671;0.27331914053646511;0.026672733875705314;0.15777077635847733;-0.42518923575613332;-0.94499203945138954;0.65962537942648047;-0.49613709851722021]
      mask Display: e = 0.06;c1 = [120 150 230]/255;c2 = ([120 150 230]+0)/383;c3 = ([120 150 230]+128)/383;patch([0 1 1 0],[0 0 1 1],c1);patch([0 1 1 1-e 1-e 0+e],[0 0 1 1-e 0+e 0+e],c2);patch([0 0 1 1-e 0+e 0+e],[0 1 1 1-e 1-e 0+e],c3);plot([0 1 1 0 0],[0 0 1 1 0]);disp('weights');
  Mux : Mux  Inputs=1
      mask Display: e = 0.06;c1 = [120 150 230]/255;c2 = ([120 150 230]+0)/383;c3 = ([120 150 230]+128)/383;patch([0 1 1 0],[0 0 1 1],c1);patch([0 1 1 1-e 1-e 0+e],[0 0 1 1-e 0+e 0+e],c2);patch([0 0 1 1-e 0+e 0+e],[0 1 1 1-e 1-e 0+e],c3);plot([0 1 1 0 0],[0 0 1 1 0]);disp('Mux');
  dotprod1 : neural/Weight Functions/dotprod  SystemSampleTime=-1
  "lz{3,2}" : Outport
      mask Display: e = 0.06;c1 = [120 230 180]/255;c2 = ([120 230 180]+0)/(256+128);c3 = ([120 230 180]+128)/(256+128);patch([0 1 1 0],[0 0 1 1],c1);patch([0 1 1 1-e 1-e 0+e],[0 0 1 1-e 0+e 0+e],c2);patch([0 0 1 1-e 0+e 0+e],[0 1 1 1-e 1-e 0+e],c3);plot([0 1 1 0 0],[0 0 1 1 0]);
  wires:
  "IW{3,2}(1,:)'"/1 -> dotprod1/1
  "ad{3,2}"/1 -> dotprod1/2
  dotprod1/1 -> Mux/1
  Mux/1 -> "lz{3,2}"/1

== system MLP_networks/net_col_c_d_4_5/Layer 1/Delays 1 ==
  "p{1}" : Inport  PortDimensions=2
      mask Display: e = 0.06;c1 = [120 230 180]/255;c2 = ([120 230 180]+0)/(256+128);c3 = ([120 230 180]+128)/(256+128);patch([0 1 1 0],[0 0 1 1],c1);patch([0 1 1 1-e 1-e 0+e],[0 0 1 1-e 0+e 0+e],c2);patch([0 0 1 1-e 0+e 0+e],[0 1 1 1-e 1-e 0+e],c3);plot([0 1 1 0 0],[0 0 1 1 0]);
  mux : Mux  Inputs=1
      mask Display: e = 0.06;c1 = [120 150 230]/255;c2 = ([120 150 230]+0)/383;c3 = ([120 150 230]+128)/383;patch([0 1 1 0],[0 0 1 1],c1);patch([0 1 1 1-e 1-e 0+e],[0 0 1 1-e 0+e 0+e],c2);patch([0 0 1 1-e 0+e 0+e],[0 1 1 1-e 1-e 0+e],c3);plot([0 1 1 0 0],[0 0 1 1 0]);disp('Mux')
  "pd{1,1}" : Outport
      mask Display: e = 0.06;c1 = [120 230 180]/255;c2 = ([120 230 180]+0)/(256+128);c3 = ([120 230 180]+128)/(256+128);patch([0 1 1 0],[0 0 1 1],c1);patch([0 1 1 1-e 1-e 0+e],[0 0 1 1-e 0+e 0+e],c2);patch([0 0 1 1-e 0+e 0+e],[0 1 1 1-e 1-e 0+e],c3);plot([0 1 1 0 0],[0 0 1 1 0]);
  wires:
  "p{1}"/1 -> mux/1
  mux/1 -> "pd{1,1}"/1
